simulink library "env_roadair_time_airConst"  (Simulink 8.7)
settings: Solver=ode45  SolverMode=SingleTasking  StartTime=0.0  StopTime=10.0  RelTol=1e-3
undefined symbols (not defined in the file): sMP
settings Model: Creator=rafrey5  LastModifiedBy=UWLELKE

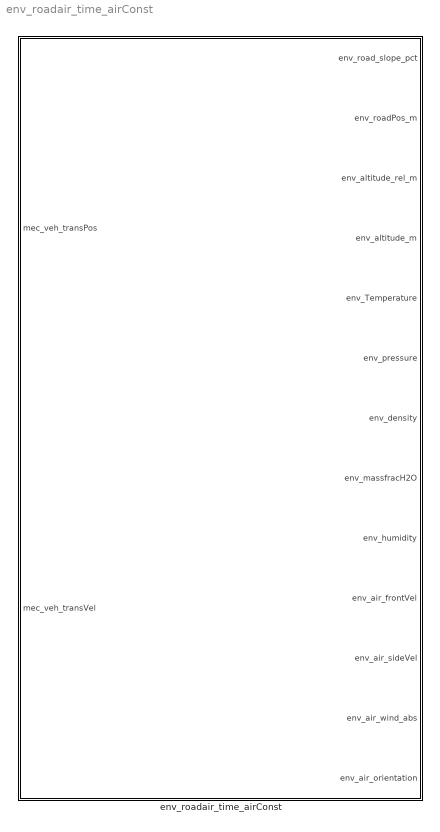
== system env_roadair_time_airConst ==
  env_roadair_time_airConst : Subsystem  TreatAsAtomicUnit=on  mask(Environment roadair implementation){CYC=sMP.bdry.env.CYC, altitude_abs_startPos_m=sMP.bdry.env.altitude_abs_startPos_m, altitude_offset_m=sMP.bdry.env.altitude_offset_m, Temperature_air_C=sMP.bdry.env.out.env_Temperature, pressure_air_mbar=sMP.bdry.env.out.env_pressure, density_air_kgm3=sMP.bdry.env.out.env_density, massfracH2O_air=sMP.bdry.env.out.env_massfracH2O, relativeHumidity_air=sMP.bdry.env.out.env_humidity, sideVel_air=sMP.bdry.env.out.env_air_sideVel, orientation_air=sMP.bdry.env.out.env_air_wind_abs, wind_abs_air=sMP.bdry.env.out.env_air_orientation}
      mask prompts: CYC "Time based Cycle Data:"; altitude_abs_startPos_m "altitude @ StartPosition [m]:"; altitude_offset_m "offset altitude [m]:"; Temperature_air_C "Air Temperature [°C]:"; pressure_air_mbar "Air pressure [mbar]:"; density_air_kgm3 "Air density [kg/m³]:"; massfracH2O_air "Air abolute humidity (water massfraction) [kg/kg]:"; relativeHumidity_air "Air relative humidity (water vapor saturation) [%]:"; sideVel_air "Side air velocity (to vehicle) [m/s]"; orientation_air "Wind orientation (over ground) [°]"; wind_abs_air "Wind velocity (over ground) [m/s]"
      mask help:
      | Generates road outputs according actual position and driver settings.
      |
      | Generates constant outputs for air properties.
      mask Help: ;

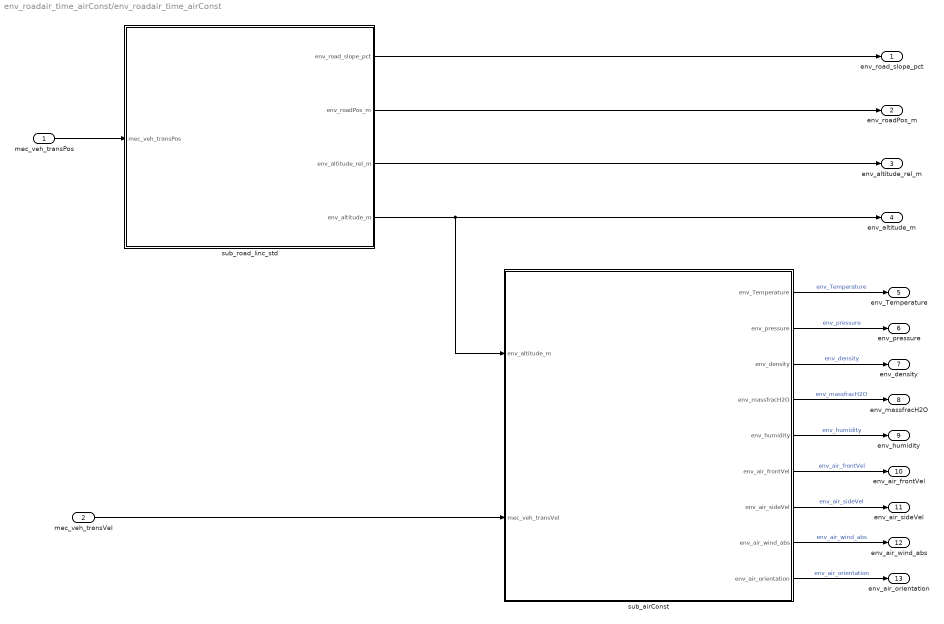
== system env_roadair_time_airConst/env_roadair_time_airConst ==
  mec_veh_transPos : Inport
  mec_veh_transVel : Inport  Port=2
  sub_airConst : Subsystem
  sub_road_linc_std : Subsystem
  env_road_slope_pct : Outport
  env_roadPos_m : Outport  Port=2
  env_altitude_rel_m : Outport  Port=3
  env_altitude_m : Outport  Port=4
  env_Temperature : Outport  Port=5
  env_pressure : Outport  Port=6
  env_density : Outport  Port=7
  env_massfracH2O : Outport  Port=8
  env_humidity : Outport  Port=9
  env_air_frontVel : Outport  Port=10
  env_air_sideVel : Outport  Port=11
  env_air_wind_abs : Outport  Port=12
  env_air_orientation : Outport  Port=13
  wires:
  sub_road_linc_std/3(env_altitude_rel_m) -> env_altitude_rel_m/1
  sub_road_linc_std/4(env_altitude_m) -> sub_airConst/1(env_altitude_m), env_altitude_m/1
  sub_road_linc_std/1(env_road_slope_pct) -> env_road_slope_pct/1
  sub_road_linc_std/2(env_roadPos_m) -> env_roadPos_m/1
  mec_veh_transPos/1 -> sub_road_linc_std/1(mec_veh_transPos)
  sub_airConst/1(env_Temperature) -> env_Temperature/1  "env_Temperature"
  sub_airConst/2(env_pressure) -> env_pressure/1  "env_pressure"
  sub_airConst/3(env_density) -> env_density/1  "env_density"
  sub_airConst/4(env_massfracH2O) -> env_massfracH2O/1  "env_massfracH2O"
  sub_airConst/5(env_humidity) -> env_humidity/1  "env_humidity"
  sub_airConst/6(env_air_frontVel) -> env_air_frontVel/1  "env_air_frontVel"
  sub_airConst/7(env_air_sideVel) -> env_air_sideVel/1  "env_air_sideVel"
  sub_airConst/8(env_air_wind_abs) -> env_air_wind_abs/1  "env_air_wind_abs"
  sub_airConst/9(env_air_orientation) -> env_air_orientation/1  "env_air_orientation"
  mec_veh_transVel/1 -> sub_airConst/2(mec_veh_transVel)

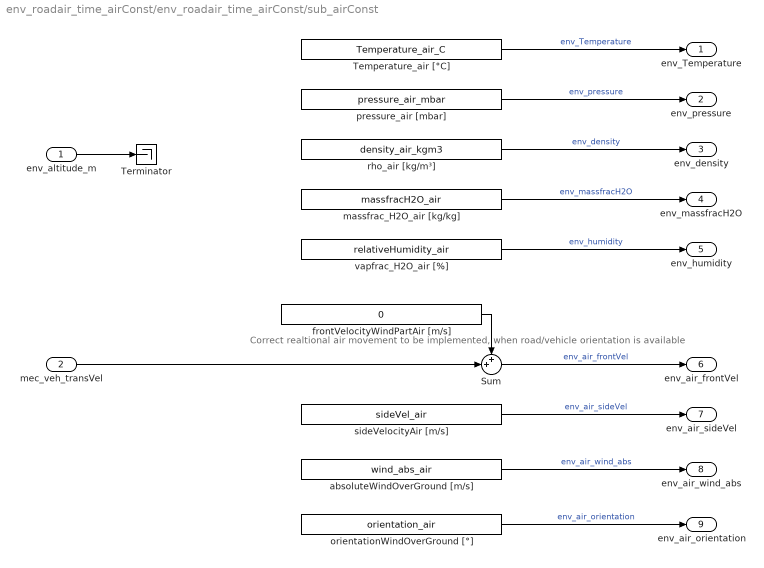
== system env_roadair_time_airConst/env_roadair_time_airConst/sub_airConst ==
  note: Correct realtional air movement to be implemented, when road/vehicle orientation is available
  env_altitude_m : Inport
  mec_veh_transVel : Inport  Port=2
  Sum : Sum  Inputs=++|
  Temperature_air [°C] : Constant  Value=Temperature_air_C
  Terminator : Terminator
  absoluteWindOverGround [m/s] : Constant  Value=wind_abs_air
  frontVelocityWindPartAir [m/s] : Constant  Value=0
  massfrac_H2O_air [kg/kg] : Constant  Value=massfracH2O_air
  orientationWindOverGround [°] : Constant  Value=orientation_air
  pressure_air [mbar] : Constant  Value=pressure_air_mbar
  rho_air [kg/m³] : Constant  Value=density_air_kgm3
  sideVelocityAir [m/s] : Constant  Value=sideVel_air
  vapfrac_H2O_air [%] : Constant  Value=relativeHumidity_air
  env_Temperature : Outport
  env_pressure : Outport  Port=2
  env_density : Outport  Port=3
  env_massfracH2O : Outport  Port=4
  env_humidity : Outport  Port=5
  env_air_frontVel : Outport  Port=6
  env_air_sideVel : Outport  Port=7
  env_air_wind_abs : Outport  Port=8
  env_air_orientation : Outport  Port=9
  wires:
  orientationWindOverGround [°]/1 -> env_air_orientation/1  "env_air_orientation"
  absoluteWindOverGround [m/s]/1 -> env_air_wind_abs/1  "env_air_wind_abs"
  sideVelocityAir [m/s]/1 -> env_air_sideVel/1  "env_air_sideVel"
  Sum/1 -> env_air_frontVel/1  "env_air_frontVel"
  env_altitude_m/1 -> Terminator/1
  vapfrac_H2O_air [%]/1 -> env_humidity/1  "env_humidity"
  massfrac_H2O_air [kg/kg]/1 -> env_massfracH2O/1  "env_massfracH2O"
  rho_air [kg/m³]/1 -> env_density/1  "env_density"
  pressure_air [mbar]/1 -> env_pressure/1  "env_pressure"
  Temperature_air [°C]/1 -> env_Temperature/1  "env_Temperature"
  frontVelocityWindPartAir [m/s]/1 -> Sum/1
  mec_veh_transVel/1 -> Sum/2

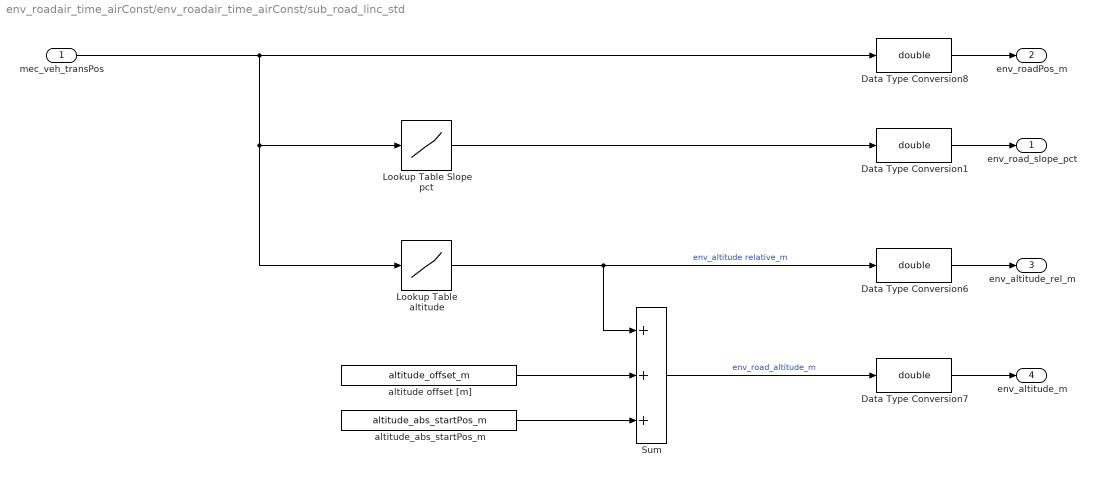
== system env_roadair_time_airConst/env_roadair_time_airConst/sub_road_linc_std ==
  mec_veh_transPos : Inport  OutDataTypeStr=double
  Data Type Conversion{1,6..8} (4 alike) : DataTypeConversion  OutDataTypeStr=double
  Lookup Table Slope pct : Lookup  InputValues=CYC.s  Table=CYC.pct_slope  LookUpMeth=Use Input Below
      settings: AttributesFormatString=|
      | Method: %<LookUpMeth>
      | [%<InputValues>; %<Table>]
  Lookup Table altitude : Lookup  InputValues=CYC.s  Table=CYC.Altitude
      settings: AttributesFormatString=|
      | Method: %<LookUpMeth>
      | [%<InputValues>; %<Table>]
  Sum : Sum  Inputs=+++
  altitude offset [m] : Constant  Value=altitude_offset_m
  altitude_abs_startPos_m : Constant  Value=altitude_abs_startPos_m
  env_road_slope_pct : Outport
  env_roadPos_m : Outport  Port=2
  env_altitude_rel_m : Outport  Port=3
  env_altitude_m : Outport  Port=4
  wires:
  altitude offset [m]/1 -> Sum/2
  Sum/1 -> Data Type Conversion7/1  "env_road_altitude_m"
  altitude_abs_startPos_m/1 -> Sum/3
  Data Type Conversion1/1 -> env_road_slope_pct/1
  Data Type Conversion6/1 -> env_altitude_rel_m/1
  Data Type Conversion7/1 -> env_altitude_m/1
  Data Type Conversion8/1 -> env_roadPos_m/1
  mec_veh_transPos/1 -> Lookup Table altitude/1, Lookup Table Slope pct/1, Data Type Conversion8/1
  Lookup Table altitude/1 -> Sum/1, Data Type Conversion6/1  "env_altitude relative_m"
  Lookup Table Slope pct/1 -> Data Type Conversion1/1
